simulink model "UE4_Demo"  (R2021a)
settings: Solver=ode14x  StartTime=0.0  StopTime=inf  FixedStep=0.01  RelTol=1e-3
libraries: simulink_extras x19, sim3dlib x18, sim3dcameralib x2
settings Model: EnablePacing=on  Creator=mojta  LastModifiedBy=mojta

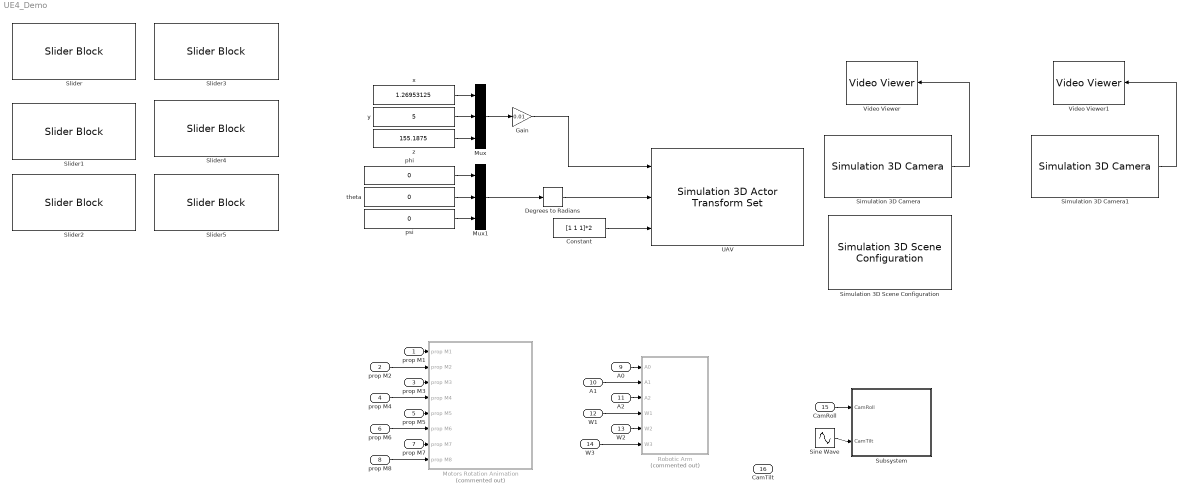
== system UE4_Demo ==
  prop M1 : Inport
  prop M2 : Inport  Port=2
  prop M3 : Inport  Port=3
  prop M4 : Inport  Port=4
  prop M5 : Inport  Port=5
  prop M6 : Inport  Port=6
  prop M7 : Inport  Port=7
  prop M8 : Inport  Port=8
  A0 : Inport  Port=9
  A1 : Inport  Port=10
  A2 : Inport  Port=11
  W1 : Inport  Port=12
  W2 : Inport  Port=13
  W3 : Inport  Port=14
  CamRoll : Inport  Port=15
  CamTilt : Inport  Port=16
  Constant : Constant  Value=[1 1 1]*2
  Degrees to Radians : simulink_extras/Transformations/Degrees to Radians
  Gain : Gain  Gain=0.01
  Motors Rotation Animation : Subsystem  Commented=on
  Mux : Mux  Inputs=3
  Mux1 : Mux  Inputs=3
  Robotic Arm : Subsystem  Commented=on
  Simulation 3D Camera : sim3dcameralib/Simulation 3D Camera  Priority=1  sensorTag=Sim3dSensor1  sensorId=1  sensorName=Sim3dSensor1  vehTagList={'Scene Origin'}  vehTag=Scene Origin  mountLoc=Origin  offsetFlag=on  tmountOffset=[0, 0, 0]  rmountOffset=[0 0 0]  FocalLength=[1109, 1109]  OpticalCenter=[640, 360]  ImageSize=[720, 1280]  RadialDistortion=[0, 0]  TangentialDistortion=[0, 0]  SensorSkew=0  DepthOutportEnabled=off  SemanticOutportEnabled=off  TransformOutportEnabled=off  SampleTime=-1  mountPoint=[0 0 0]  mountOrientation=[0 0 0]  aMode=3  ID=1
      settings: SourceProductBaseCode=DR,UV,VE
  Simulation 3D Camera1 : sim3dcameralib/Simulation 3D Camera  Priority=1  sensorTag=Sim3dSensor2  sensorId=2  sensorName=Sim3dSensor2  vehTagList={'Scene Origin'}  vehTag=Scene Origin  mountLoc=Origin  offsetFlag=on  tmountOffset=[0, 0, 0]  rmountOffset=[0 0 90]  FocalLength=[1109, 1109]  OpticalCenter=[640, 360]  ImageSize=[720, 1280]  RadialDistortion=[0, 0]  TangentialDistortion=[0, 0]  SensorSkew=0  DepthOutportEnabled=off  SemanticOutportEnabled=off  TransformOutportEnabled=off  SampleTime=-1  mountPoint=[0 0 0]  mountOrientation=[0 0 -90]  aMode=3  ID=2
      settings: SourceProductBaseCode=DR,UV,VE
  Simulation 3D Scene Configuration : sim3dlib/Simulation 3D Scene Configuration  Priority=0  ProjectFormat=Unreal Editor  SceneDesc=Straight road  ProjectName=C:\Program Files\Polyspace\R2021a\toolbox\shared\sim3d_projects\automotive_project\UE4\WindowsNoEditor\VehicleSimulation.exe  ScenePath=/Game/Maps/HwStrght  UEProjPath=D:\MS_Control_Project\Sim_Env\Environment_1\Environment_1.uproject  vehTagList={'Scene Origin'}  vehTag=Scene Origin  OpVisEn=off  Ts=0.02  EnableWindow=on  EnableWeather=off  SunAltitude=40.0  SunAzimuth=90  clouds=10  wind=1  fog=0  rain=0  sensorTag=MainCamera2  sensorId=2  sensorName=MainCamera2  mountLoc=Origin  offsetFlag=off  tmountOffset=[0, 0, 0]  rmountOffset=[0, 0, 0]  HorizontalResolution=1280  VerticalResolution=720  HorizontalFOV=60  mountPoint=[0 0 0]  mountOrientation=[0 0 0]  aMode=2  ID=2
      settings: SourceProductBaseCode=DR,UV,VE
  Sine Wave : Sin  Amplitude=90  SampleTime=0
  Slider : SliderBlock  ScaleMin=-200  ScaleMax=200
  Slider1 : SliderBlock  ScaleMin=-200  ScaleMax=200
  Slider2 : SliderBlock  ScaleMin=20  ScaleMax=300
  Slider3 : SliderBlock  ScaleMin=-30  ScaleMax=30  TickInterval=10
  Slider4 : SliderBlock  ScaleMin=-30  ScaleMax=30  TickInterval=10
  Slider5 : SliderBlock  ScaleMin=-30  ScaleMax=30  TickInterval=10
  Subsystem : Subsystem
  UAV : sim3dlib/Simulation 3D Actor Transform Set  Priority=-1  ActorTag=uav  NumberOfParts=1  CustNumOfParts=3  Translation=[0 0 0]  Rotation=[0 0 0]  Scale=[1 1 1]  Ts=-1  aMode=2
      settings: SourceProductBaseCode=DR,UV,VE
  Video Viewer : VideoViewer  FigPos=[83 1018 1426 783]
  Video Viewer1 : VideoViewer  FigPos=[191 986 1426 783]
  phi : Constant  Value=0
  psi : Constant  Value=0
  theta : Constant  Value=0
  x : Constant  Value=1.26953125
  y : Constant  Value=5
  z : Constant  Value=155.1875
  wires:
  Constant/1 -> UAV/3
  Mux1/1 -> Degrees to Radians/1
  Mux/1 -> Gain/1
  x/1 -> Mux/1
  y/1 -> Mux/2
  z/1 -> Mux/3
  psi/1 -> Mux1/3
  theta/1 -> Mux1/2
  phi/1 -> Mux1/1
  Degrees to Radians/1 -> UAV/2
  Gain/1 -> UAV/1
  Simulation 3D Camera/1 -> Video Viewer/1
  prop M1/1 -> Motors Rotation Animation/1(prop M1)
  prop M2/1 -> Motors Rotation Animation/2(prop M2)
  prop M3/1 -> Motors Rotation Animation/3(prop M3)
  prop M4/1 -> Motors Rotation Animation/4(prop M4)
  prop M5/1 -> Motors Rotation Animation/5(prop M5)
  prop M6/1 -> Motors Rotation Animation/6(prop M6)
  prop M7/1 -> Motors Rotation Animation/7(prop M7)
  prop M8/1 -> Motors Rotation Animation/8(prop M8)
  A1/1 -> Robotic Arm/2(A1)
  A2/1 -> Robotic Arm/3(A2)
  W1/1 -> Robotic Arm/4(W1)
  W2/1 -> Robotic Arm/5(W2)
  W3/1 -> Robotic Arm/6(W3)
  A0/1 -> Robotic Arm/1(A0)
  CamRoll/1 -> Subsystem/1(CamRoll)
  Sine Wave/1 -> Subsystem/2(CamTilt)
  Simulation 3D Camera1/1 -> Video Viewer1/1

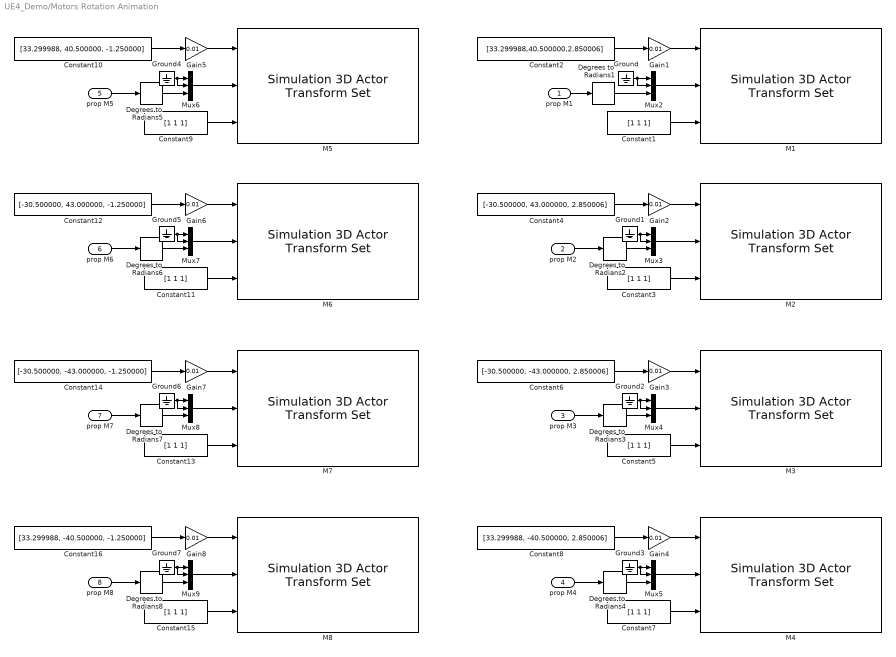
== system UE4_Demo/Motors Rotation Animation ==
  prop M1 : Inport
  prop M2 : Inport  Port=2
  prop M3 : Inport  Port=3
  prop M4 : Inport  Port=4
  prop M5 : Inport  Port=5
  prop M6 : Inport  Port=6
  prop M7 : Inport  Port=7
  prop M8 : Inport  Port=8
  Constant{1,3,5,7,9,11,13,15} (8 alike) : Constant  Value=[1 1 1]
  Constant10 : Constant  Value=[33.299988, 40.500000, -1.250000]
  Constant12 : Constant  Value=[-30.500000, 43.000000, -1.250000]
  Constant14 : Constant  Value=[-30.500000, -43.000000, -1.250000]
  Constant16 : Constant  Value=[33.299988, -40.500000, -1.250000]
  Constant2 : Constant  Value=[33.299988,40.500000,2.850006]
  Constant4 : Constant  Value=[-30.500000, 43.000000, 2.850006]
  Constant6 : Constant  Value=[-30.500000, -43.000000, 2.850006]
  Constant8 : Constant  Value=[33.299988, -40.500000, 2.850006]
  Degrees to Radians{1..8} (8 alike) : simulink_extras/Transformations/Degrees to Radians
  Gain{1..8} (8 alike) : Gain  Gain=0.01
  Ground{,1..7} (8 alike) : Ground
  M1 : sim3dlib/Simulation 3D Actor Transform Set  Priority=-1  ActorTag=M1  NumberOfParts=1  CustNumOfParts=3  Translation=[0 0 0]  Rotation=[0 0 0]  Scale=[1 1 1]  Ts=-1  aMode=2
      settings: SourceProductBaseCode=DR,UV,VE
  M2 : sim3dlib/Simulation 3D Actor Transform Set  Priority=-1  ActorTag=M2  NumberOfParts=1  CustNumOfParts=3  Translation=[0 0 0]  Rotation=[0 0 0]  Scale=[1 1 1]  Ts=-1  aMode=2
      settings: SourceProductBaseCode=DR,UV,VE
  M3 : sim3dlib/Simulation 3D Actor Transform Set  Priority=-1  ActorTag=M3  NumberOfParts=1  CustNumOfParts=3  Translation=[0 0 0]  Rotation=[0 0 0]  Scale=[1 1 1]  Ts=-1  aMode=2
      settings: SourceProductBaseCode=DR,UV,VE
  M4 : sim3dlib/Simulation 3D Actor Transform Set  Priority=-1  ActorTag=M4  NumberOfParts=1  CustNumOfParts=3  Translation=[0 0 0]  Rotation=[0 0 0]  Scale=[1 1 1]  Ts=-1  aMode=2
      settings: SourceProductBaseCode=DR,UV,VE
  M5 : sim3dlib/Simulation 3D Actor Transform Set  Priority=-1  ActorTag=M5  NumberOfParts=1  CustNumOfParts=3  Translation=[0 0 0]  Rotation=[0 0 0]  Scale=[1 1 1]  Ts=-1  aMode=2
      settings: SourceProductBaseCode=DR,UV,VE
  M6 : sim3dlib/Simulation 3D Actor Transform Set  Priority=-1  ActorTag=M6  NumberOfParts=1  CustNumOfParts=3  Translation=[0 0 0]  Rotation=[0 0 0]  Scale=[1 1 1]  Ts=-1  aMode=2
      settings: SourceProductBaseCode=DR,UV,VE
  M7 : sim3dlib/Simulation 3D Actor Transform Set  Priority=-1  ActorTag=M7  NumberOfParts=1  CustNumOfParts=3  Translation=[0 0 0]  Rotation=[0 0 0]  Scale=[1 1 1]  Ts=-1  aMode=2
      settings: SourceProductBaseCode=DR,UV,VE
  M8 : sim3dlib/Simulation 3D Actor Transform Set  Priority=-1  ActorTag=M8  NumberOfParts=1  CustNumOfParts=3  Translation=[0 0 0]  Rotation=[0 0 0]  Scale=[1 1 1]  Ts=-1  aMode=2
      settings: SourceProductBaseCode=DR,UV,VE
  Mux{2..9} (8 alike) : Mux  Inputs=3
  wires:
  Ground7/1 -> Mux9/1, Mux9/2
  Mux9/1 -> M8/2
  Constant7/1 -> M4/3
  Constant1/1 -> M1/3
  Gain8/1 -> M8/1
  Constant15/1 -> M8/3
  Constant16/1 -> Gain8/1
  Ground5/1 -> Mux7/2, Mux7/1
  prop M5/1 -> Degrees to Radians5/1
  Constant12/1 -> Gain6/1
  Constant6/1 -> Gain3/1
  prop M7/1 -> Degrees to Radians7/1
  Degrees to Radians1/1 -> Mux2/3
  Mux5/1 -> M4/2
  prop M2/1 -> Degrees to Radians2/1
  prop M4/1 -> Degrees to Radians4/1
  Gain7/1 -> M7/1
  Constant11/1 -> M6/3
  Degrees to Radians7/1 -> Mux8/3
  Mux8/1 -> M7/2
  Degrees to Radians6/1 -> Mux7/3
  Constant5/1 -> M3/3
  Mux4/1 -> M3/2
  Constant13/1 -> M7/3
  Gain1/1 -> M1/1
  Mux7/1 -> M6/2
  prop M3/1 -> Degrees to Radians3/1
  Constant14/1 -> Gain7/1
  prop M6/1 -> Degrees to Radians6/1
  Mux6/1 -> M5/2
  Gain6/1 -> M6/1
  Gain5/1 -> M5/1
  Degrees to Radians5/1 -> Mux6/3
  Degrees to Radians2/1 -> Mux3/3
  Gain3/1 -> M3/1
  Constant10/1 -> Gain5/1
  Constant8/1 -> Gain4/1
  Constant9/1 -> M5/3
  Constant4/1 -> Gain2/1
  Ground1/1 -> Mux3/2, Mux3/1
  Ground6/1 -> Mux8/1, Mux8/2
  Constant2/1 -> Gain1/1
  Ground4/1 -> Mux6/2, Mux6/1
  Ground3/1 -> Mux5/2, Mux5/1
  Ground/1 -> Mux2/2, Mux2/1
  Constant3/1 -> M2/3
  Ground2/1 -> Mux4/2, Mux4/1
  prop M8/1 -> Degrees to Radians8/1
  Mux3/1 -> M2/2
  Gain2/1 -> M2/1
  prop M1/1 -> Degrees to Radians1/1
  Mux2/1 -> M1/2
  Gain4/1 -> M4/1
  Degrees to Radians8/1 -> Mux9/3
  Degrees to Radians3/1 -> Mux4/3
  Degrees to Radians4/1 -> Mux5/3

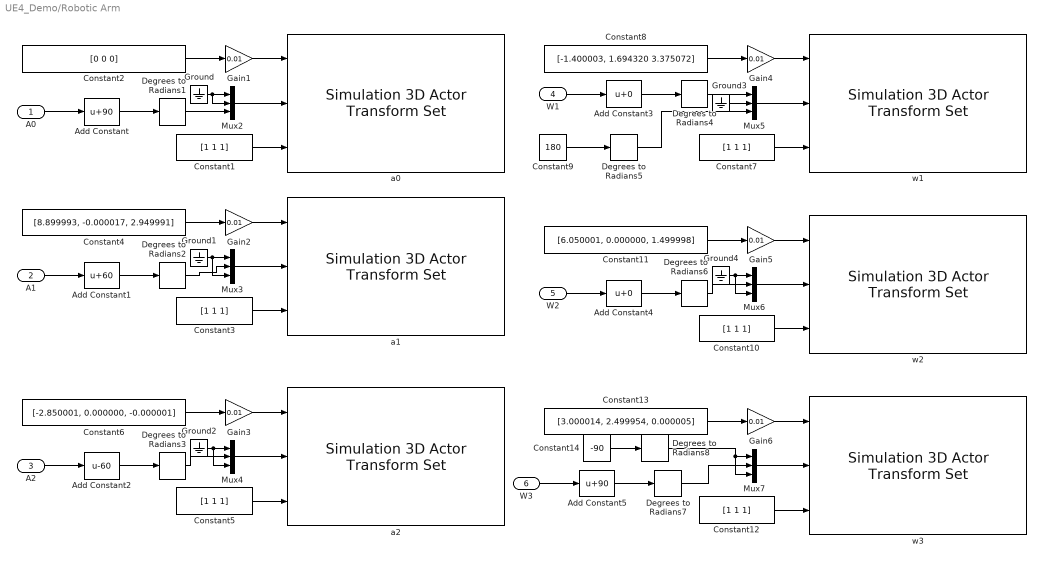
== system UE4_Demo/Robotic Arm ==
  A0 : Inport
  A1 : Inport  Port=2
  A2 : Inport  Port=3
  W1 : Inport  Port=4
  W2 : Inport  Port=5
  W3 : Inport  Port=6
  Add Constant : Bias  Bias=90
  Add Constant1 : Bias  Bias=60
  Add Constant2 : Bias  Bias=-60
  Add Constant3 : Bias
  Add Constant4 : Bias
  Add Constant5 : Bias  Bias=90
  Constant{1,3,5,7,10,12} (6 alike) : Constant  Value=[1 1 1]
  Constant11 : Constant  Value=[6.050001, 0.000000, 1.499998]
  Constant13 : Constant  Value=[3.000014, 2.499954, 0.000005]
  Constant14 : Constant  Value=-90
  Constant2 : Constant  Value=[0 0 0]
  Constant4 : Constant  Value=[8.899993, -0.000017, 2.949991]
  Constant6 : Constant  Value=[-2.850001, 0.000000, -0.000001]
  Constant8 : Constant  Value=[-1.400003, 1.694320 3.375072]
  Constant9 : Constant  Value=180
  Degrees to Radians{1..8} (8 alike) : simulink_extras/Transformations/Degrees to Radians
  Gain{1..6} (6 alike) : Gain  Gain=0.01
  Ground{,1..4} (5 alike) : Ground
  Mux{2..7} (6 alike) : Mux  Inputs=3
  a0 : sim3dlib/Simulation 3D Actor Transform Set  Priority=-1  ActorTag=A0  NumberOfParts=1  CustNumOfParts=3  Translation=[0 0 0]  Rotation=[0 0 0]  Scale=[1 1 1]  Ts=-1  aMode=2
      settings: SourceProductBaseCode=DR,UV,VE
  a1 : sim3dlib/Simulation 3D Actor Transform Set  Priority=-1  ActorTag=A1  NumberOfParts=1  CustNumOfParts=3  Translation=[0 0 0]  Rotation=[0 0 0]  Scale=[1 1 1]  Ts=-1  aMode=2
      settings: SourceProductBaseCode=DR,UV,VE
  a2 : sim3dlib/Simulation 3D Actor Transform Set  Priority=-1  ActorTag=A2  NumberOfParts=1  CustNumOfParts=3  Translation=[0 0 0]  Rotation=[0 0 0]  Scale=[1 1 1]  Ts=-1  aMode=2
      settings: SourceProductBaseCode=DR,UV,VE
  w1 : sim3dlib/Simulation 3D Actor Transform Set  Priority=-1  ActorTag=W1  NumberOfParts=1  CustNumOfParts=3  Translation=[0 0 0]  Rotation=[0 0 0]  Scale=[1 1 1]  Ts=-1  aMode=2
      settings: SourceProductBaseCode=DR,UV,VE
  w2 : sim3dlib/Simulation 3D Actor Transform Set  Priority=-1  ActorTag=W2  NumberOfParts=1  CustNumOfParts=3  Translation=[0 0 0]  Rotation=[0 0 0]  Scale=[1 1 1]  Ts=-1  aMode=2
      settings: SourceProductBaseCode=DR,UV,VE
  w3 : sim3dlib/Simulation 3D Actor Transform Set  Priority=-1  ActorTag=W3  NumberOfParts=1  CustNumOfParts=3  Translation=[0 0 0]  Rotation=[0 0 0]  Scale=[1 1 1]  Ts=-1  aMode=2
      settings: SourceProductBaseCode=DR,UV,VE
  wires:
  Constant7/1 -> w1/3
  Degrees to Radians2/1 -> Mux3/2
  W1/1 -> Add Constant3/1
  Mux3/1 -> a1/2
  Ground3/1 -> Mux5/2
  Constant14/1 -> Degrees to Radians8/1
  Gain4/1 -> w1/1
  Constant9/1 -> Degrees to Radians5/1
  Ground/1 -> Mux2/2, Mux2/1
  Degrees to Radians4/1 -> Mux5/1
  Constant8/1 -> Gain4/1
  Add Constant3/1 -> Degrees to Radians4/1
  Mux5/1 -> w1/2
  Mux7/1 -> w3/2
  Constant2/1 -> Gain1/1
  Degrees to Radians8/1 -> Mux7/1, Mux7/3
  Degrees to Radians1/1 -> Mux2/3
  Add Constant/1 -> Degrees to Radians1/1
  Constant1/1 -> a0/3
  Constant5/1 -> a2/3
  Mux6/1 -> w2/2
  Constant6/1 -> Gain3/1
  Mux2/1 -> a0/2
  Gain1/1 -> a0/1
  W2/1 -> Add Constant4/1
  Ground4/1 -> Mux6/3, Mux6/1
  Constant4/1 -> Gain2/1
  Constant11/1 -> Gain5/1
  Constant3/1 -> a1/3
  Add Constant4/1 -> Degrees to Radians6/1
  Mux4/1 -> a2/2
  Constant12/1 -> w3/3
  Degrees to Radians7/1 -> Mux7/2
  Constant13/1 -> Gain6/1
  W3/1 -> Add Constant5/1
  Add Constant2/1 -> Degrees to Radians3/1
  Gain6/1 -> w3/1
  Add Constant5/1 -> Degrees to Radians7/1
  A0/1 -> Add Constant/1
  Degrees to Radians3/1 -> Mux4/2
  A2/1 -> Add Constant2/1
  Gain5/1 -> w2/1
  Add Constant1/1 -> Degrees to Radians2/1
  Constant10/1 -> w2/3
  Gain2/1 -> a1/1
  Ground1/1 -> Mux3/3, Mux3/1
  Degrees to Radians5/1 -> Mux5/3
  Ground2/1 -> Mux4/3, Mux4/1
  Gain3/1 -> a2/1
  A1/1 -> Add Constant1/1
  Degrees to Radians6/1 -> Mux6/2

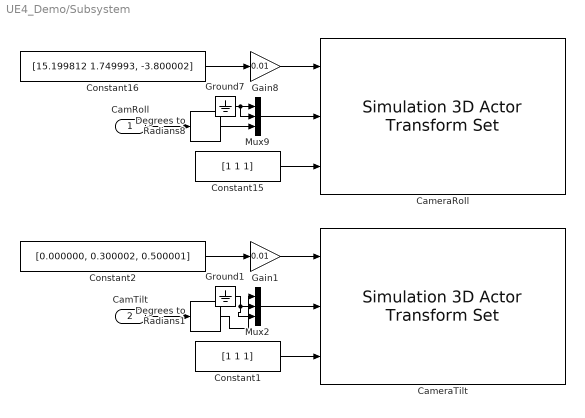
== system UE4_Demo/Subsystem ==
  CamRoll : Inport
  CamTilt : Inport  Port=2
  CameraRoll : sim3dlib/Simulation 3D Actor Transform Set  Priority=-1  ActorTag=CamRoll  NumberOfParts=1  CustNumOfParts=3  Translation=[0 0 0]  Rotation=[0 0 0]  Scale=[1 1 1]  Ts=-1  aMode=2
      settings: SourceProductBaseCode=DR,UV,VE
  CameraTilt : sim3dlib/Simulation 3D Actor Transform Set  Priority=-1  ActorTag=CamTilt  NumberOfParts=1  CustNumOfParts=3  Translation=[0 0 0]  Rotation=[0 0 0]  Scale=[1 1 1]  Ts=-1  aMode=2
      settings: SourceProductBaseCode=DR,UV,VE
  Constant1 : Constant  Value=[1 1 1]
  Constant15 : Constant  Value=[1 1 1]
  Constant16 : Constant  Value=[15.199812 1.749993, -3.800002]
  Constant2 : Constant  Value=[0.000000, 0.300002, 0.500001]
  Degrees to Radians1 : simulink_extras/Transformations/Degrees to Radians
  Degrees to Radians8 : simulink_extras/Transformations/Degrees to Radians
  Gain1 : Gain  Gain=0.01
  Gain8 : Gain  Gain=0.01
  Ground1 : Ground
  Ground7 : Ground
  Mux2 : Mux  Inputs=3
  Mux9 : Mux  Inputs=3
  wires:
  Gain1/1 -> CameraTilt/1
  Constant15/1 -> CameraRoll/3
  Constant16/1 -> Gain8/1
  Ground1/1 -> Mux2/2, Mux2/3
  Gain8/1 -> CameraRoll/1
  Constant1/1 -> CameraTilt/3
  Ground7/1 -> Mux9/1, Mux9/2
  Degrees to Radians8/1 -> Mux9/3
  Mux9/1 -> CameraRoll/2
  CamRoll/1 -> Degrees to Radians8/1
  CamTilt/1 -> Degrees to Radians1/1
  Constant2/1 -> Gain1/1
  Mux2/1 -> CameraTilt/2
  Degrees to Radians1/1 -> Mux2/1
